simulink model "autotest"  (R2017b)
settings: Solver=VariableStepAuto  StartTime=20  StopTime=200  RelTol=1e-3
settings Model: Creator=Administrator  LastModifiedBy=Administrator
settings DataIOCC: SaveFormat=Array

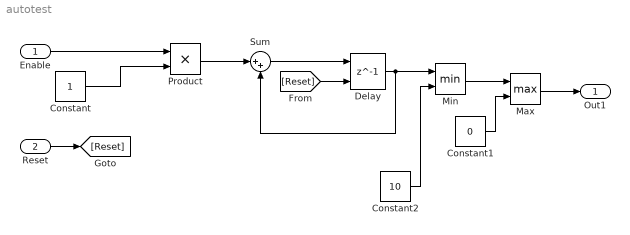
== system autotest ==
  Enable : Inport
  "Reset " : Inport  Port=2
  Constant : Constant
  Constant1 : Constant  Value=0
  Constant2 : Constant  Value=10
  Delay : Delay  DelayLength=1  ExternalReset=Level
      settings: InputPortMap=u0,r5
  Max : MinMax  Function=max  Inputs=2
  Min : MinMax  Inputs=2
  Product : Product
  Sum : Sum  Inputs=|++
  Out1 : Outport
  wires:
  Enable/1 -> Product/1
  Constant/1 -> Product/2
  Product/1 -> Sum/1
  Sum/1 -> Delay/1
  Min/1 -> Max/1
  Delay/1 -> Sum/2, Min/1
  Max/1 -> Out1/1
  Constant1/1 -> Max/2
  Constant2/1 -> Min/2
  "Reset "/1 -> [Reset]
  [Reset] -> Delay/2
